simulink model "pmnl1"  (R2018a)
settings: Solver=VariableStepAuto  StartTime=0.0  StopTime=0.5  RelTol=1e-3
settings Model: Creator=pc  LastModifiedBy=pc

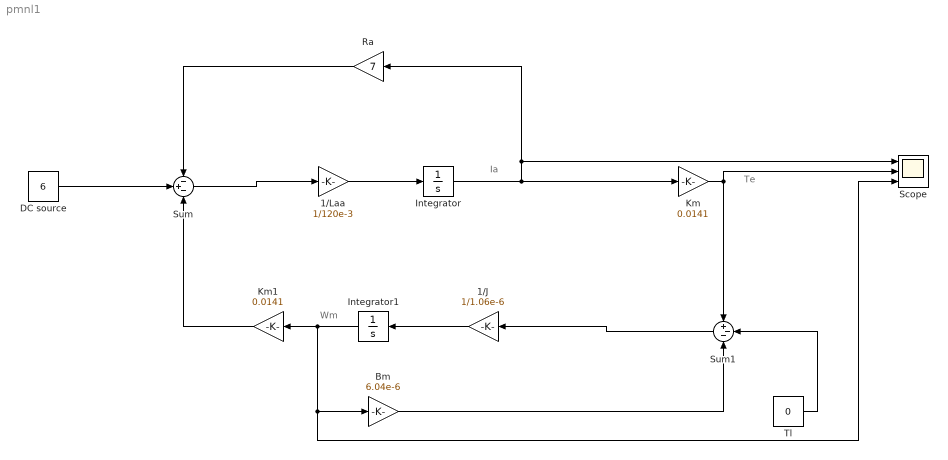
== system pmnl1 ==
  note: Wm
  note: Te
  note: Ia
  1/J : Gain  Gain=1/1.06e-6
  1/Laa : Gain  Gain=1/120e-3
  Bm : Gain  Gain=6.04e-6
  DC source : Constant  Value=6
  Integrator : Integrator
  Integrator1 : Integrator
  Km : Gain  Gain=0.0141
  Km1 : Gain  Gain=0.0141
  Ra : Gain  Gain=7
  Scope : Scope  NumInputPorts=3
  Sum : Sum  Inputs=-+-
  Sum1 : Sum  Inputs=+--
  Tl : Constant  Value=0
  wires:
  DC source/1 -> Sum/2
  Sum/1 -> 1/Laa/1
  Ra/1 -> Sum/1
  1/Laa/1 -> Integrator/1
  Integrator/1 -> Scope/1, Ra/1, Km/1
  Km/1 -> Sum1/1, Scope/2
  Tl/1 -> Sum1/2
  Bm/1 -> Sum1/3
  Sum1/1 -> 1/J/1
  1/J/1 -> Integrator1/1
  Integrator1/1 -> Km1/1, Scope/3, Bm/1
  Km1/1 -> Sum/3
